simulink model "addTw_mdl5"  (R2014a)
settings: Solver=FixedStepDiscrete  SolverMode=SingleTasking  StartTime=TIME(1)  StopTime=TIME(end)  FixedStep=SIMSTEP  RelTol=1e-3
model workspace (MAT data in the model file):
  autoc_mdd_data01 : struct (value not decoded)
undefined symbols (not defined in the file or in its folder): map_mr4_01, map_mr4_02, map_mr4_03, map_mr4_04, map_mr4_05, map_mr4_06, map_mr4_07, map_mr4_08, Parameter114, Parameter115, Parameter131, Parameter141, Parameter143, Parameter144, Parameter51, Parameter52, Parameter53, Parameter70, Parameter71, Parameter92, Parameter93, SIMSTEP
(part 3 of 3)

== system addTw_mdl5/SubSystem2611/SubSystem2691/SubSystem2693/SubSystem2695/SubSystem2703 ==
  note: ***編集禁止***
  input : Inport
  element : Inport  Port=2
  Assignment : Assignment  IndexOptions=Index vector (port)  OutputSizes=[1 1]
  Inside_DSR : DataStoreRead  DataStoreName=DSM335
  Inside_DSW : DataStoreWrite  DataStoreName=DSM335
  wires:
  element/1 -> Assignment/3
  input/1 -> Assignment/2
  Inside_DSR/1 -> Assignment/1
  Assignment/1 -> Inside_DSW/1

== system addTw_mdl5/SubSystem2611/SubSystem2691/SubSystem2693/SubSystem2695/SubSystem2704 ==
  note: ***編集禁止***
  input : Inport
  element : Inport  Port=2
  Assignment : Assignment  IndexOptions=Index vector (port)  OutputSizes=[1 1]
  Inside_DSR : DataStoreRead  DataStoreName=DSM348
  Inside_DSW : DataStoreWrite  DataStoreName=DSM348
  wires:
  Assignment/1 -> Inside_DSW/1
  Inside_DSR/1 -> Assignment/1
  input/1 -> Assignment/2
  element/1 -> Assignment/3

== system addTw_mdl5/SubSystem2611/SubSystem2691/SubSystem2693/SubSystem2695/SubSystem2705 ==
  note: ***編集禁止***
  input : Inport
  element : Inport  Port=2
  Assignment : Assignment  IndexOptions=Index vector (port)  OutputSizes=[1 1]
  Inside_DSR : DataStoreRead  DataStoreName=DSM349
  Inside_DSW : DataStoreWrite  DataStoreName=DSM349
  wires:
  Assignment/1 -> Inside_DSW/1
  Inside_DSR/1 -> Assignment/1
  input/1 -> Assignment/2
  element/1 -> Assignment/3

== system addTw_mdl5/SubSystem2611/SubSystem2691/SubSystem2693/SubSystem2695/SubSystem2706 ==
  note: ***編集禁止***
  input : Inport
  element : Inport  Port=2
  Assignment : Assignment  IndexOptions=Index vector (port)  OutputSizes=[1 1]
  Inside_DSR : DataStoreRead  DataStoreName=DSM347
  Inside_DSW : DataStoreWrite  DataStoreName=DSM347
  wires:
  Assignment/1 -> Inside_DSW/1
  Inside_DSR/1 -> Assignment/1
  input/1 -> Assignment/2
  element/1 -> Assignment/3

== system addTw_mdl5/SubSystem2611/SubSystem2612/SubSystem2620/SubSystem2624/SubSystem2627/SubSystem2628 ==
  note: ***編集禁止***
  element : Inport
  Inside_DSR : DataStoreRead  DataStoreName=DSM147
  Selector : Selector  IndexOptions=Index vector (port)  Indices=[1 3]
  Output : Outport
  wires:
  Selector/1 -> Output/1
  element/1 -> Selector/2
  Inside_DSR/1 -> Selector/1

== system addTw_mdl5/SubSystem2611/SubSystem2612/SubSystem2620/SubSystem2624/SubSystem2627/SubSystem2629 ==
  note: ***編集禁止***
  element : Inport
  Inside_DSR : DataStoreRead  DataStoreName=DSM304
  Selector : Selector  IndexOptions=Index vector (port)  Indices=[1 3]
  Output : Outport
  wires:
  Inside_DSR/1 -> Selector/1
  element/1 -> Selector/2
  Selector/1 -> Output/1

== system addTw_mdl5/SubSystem2611/SubSystem2612/SubSystem2620/SubSystem2624/SubSystem2627/SubSystem2630 ==
  note: ***編集禁止***
  element : Inport
  Inside_DSR : DataStoreRead  DataStoreName=DSM346
  Selector : Selector  IndexOptions=Index vector (port)  Indices=[1 3]
  Output : Outport
  wires:
  Selector/1 -> Output/1
  element/1 -> Selector/2
  Inside_DSR/1 -> Selector/1

== system addTw_mdl5/SubSystem2611/SubSystem2612/SubSystem2620/SubSystem2624/SubSystem2627/SubSystem2631 ==
  note: ***編集禁止***
  input : Inport
  element : Inport  Port=2
  Assignment : Assignment  IndexOptions=Index vector (port)  OutputSizes=[1 1]
  Inside_DSR : DataStoreRead  DataStoreName=DSM346
  Inside_DSW : DataStoreWrite  DataStoreName=DSM346
  wires:
  Assignment/1 -> Inside_DSW/1
  Inside_DSR/1 -> Assignment/1
  input/1 -> Assignment/2
  element/1 -> Assignment/3

== system addTw_mdl5/SubSystem2611/SubSystem2612/SubSystem2620/SubSystem2624/SubSystem2627/SubSystem2632 ==
  note: ***編集禁止***
  input : Inport
  element : Inport  Port=2
  Assignment : Assignment  IndexOptions=Index vector (port)  OutputSizes=[1 1]
  Inside_DSR : DataStoreRead  DataStoreName=DSM349
  Inside_DSW : DataStoreWrite  DataStoreName=DSM349
  wires:
  Assignment/1 -> Inside_DSW/1
  Inside_DSR/1 -> Assignment/1
  input/1 -> Assignment/2
  element/1 -> Assignment/3

== system addTw_mdl5/SubSystem2611/SubSystem2612/SubSystem2620/SubSystem2624/SubSystem2627/SubSystem2633 ==
  note: ***編集禁止***
  input : Inport
  element : Inport  Port=2
  Assignment : Assignment  IndexOptions=Index vector (port)  OutputSizes=[1 1]
  Inside_DSR : DataStoreRead  DataStoreName=DSM348
  Inside_DSW : DataStoreWrite  DataStoreName=DSM348
  wires:
  element/1 -> Assignment/3
  input/1 -> Assignment/2
  Inside_DSR/1 -> Assignment/1
  Assignment/1 -> Inside_DSW/1

== system addTw_mdl5/SubSystem2611/SubSystem2612/SubSystem2620/SubSystem2624/SubSystem2627/SubSystem2634 ==
  note: ***編集禁止***
  input : Inport
  element : Inport  Port=2
  Assignment : Assignment  IndexOptions=Index vector (port)  OutputSizes=[1 1]
  Inside_DSR : DataStoreRead  DataStoreName=DSM347
  Inside_DSW : DataStoreWrite  DataStoreName=DSM347
  wires:
  element/1 -> Assignment/3
  input/1 -> Assignment/2
  Inside_DSR/1 -> Assignment/1
  Assignment/1 -> Inside_DSW/1

== system addTw_mdl5/SubSystem2611/SubSystem2612/SubSystem2620/SubSystem2624/SubSystem2627/SubSystem2635 ==
  note: ***編集禁止***
  In1 : Inport
  In2 : Inport  Port=2
  RO1 : RelationalOperator  Operator===  InputSameDT=on
  single1 : DataTypeConversion  OutDataTypeStr=single  SaturateOnIntegerOverflow=on  RndMeth=Zero
  single2 : DataTypeConversion  OutDataTypeStr=single  SaturateOnIntegerOverflow=on  RndMeth=Zero
  Out1 : Outport
  wires:
  single2/1 -> RO1/2
  single1/1 -> RO1/1
  In1/1 -> single1/1
  In2/1 -> single2/1
  RO1/1 -> Out1/1

== system addTw_mdl5/SubSystem2611/SubSystem2612/SubSystem2620/SubSystem2624/SubSystem2638/SubSystem2639 ==
  note: ***編集禁止***
  element : Inport
  Inside_DSR : DataStoreRead  DataStoreName=DSM97
  Selector : Selector  IndexOptions=Index vector (port)  Indices=[1 3]
  Output : Outport
  wires:
  Inside_DSR/1 -> Selector/1
  element/1 -> Selector/2
  Selector/1 -> Output/1

== system addTw_mdl5/SubSystem2611/SubSystem2612/SubSystem2620/SubSystem2624/SubSystem2638/SubSystem2640 ==
  note: ***編集禁止***
  element : Inport
  Inside_DSR : DataStoreRead  DataStoreName=DSM318
  Selector : Selector  IndexOptions=Index vector (port)  Indices=[1 3]
  Output : Outport
  wires:
  Selector/1 -> Output/1
  element/1 -> Selector/2
  Inside_DSR/1 -> Selector/1

== system addTw_mdl5/SubSystem2611/SubSystem2612/SubSystem2620/SubSystem2624/SubSystem2638/SubSystem2641 ==
  note: ***編集禁止***
  mult : Inport
  div : Inport  Port=2
  Product : Product  Inputs=*/  SaturateOnIntegerOverflow=on  RndMeth=Zero  InputSameDT=on  OutDataTypeStr=Inherit: Same as first input
  Out : Outport
  wires:
  div/1 -> Product/2
  mult/1 -> Product/1
  Product/1 -> Out/1

== system addTw_mdl5/SubSystem2611/SubSystem2612/SubSystem2620/SubSystem2624/SubSystem2638/SubSystem2642 ==
  note: ***編集禁止***
  mult : Inport
  div : Inport  Port=2
  Product : Product  Inputs=*/  SaturateOnIntegerOverflow=on  RndMeth=Zero  InputSameDT=on  OutDataTypeStr=Inherit: Same as first input
  Out : Outport
  wires:
  Product/1 -> Out/1
  mult/1 -> Product/1
  div/1 -> Product/2

== system addTw_mdl5/SubSystem2611/SubSystem2612/SubSystem2620/SubSystem2624/SubSystem2638/SubSystem2643 ==
  note: ***編集禁止***
  Max : Inport
  Input : Inport  Port=2
  Min1 : MinMax  Inputs=2  SaturateOnIntegerOverflow=on  InputSameDT=on
  Output : Outport
  wires:
  Max/1 -> Min1/1
  Input/1 -> Min1/2
  Min1/1 -> Output/1

== system addTw_mdl5/SubSystem2611/SubSystem2612/SubSystem2620/SubSystem2624/SubSystem2644/SubSystem2645 ==
  note: ***編集禁止***
  element : Inport
  Inside_DSR : DataStoreRead  DataStoreName=DSM115
  Selector : Selector  IndexOptions=Index vector (port)  Indices=[1 3]
  Output : Outport
  wires:
  Inside_DSR/1 -> Selector/1
  element/1 -> Selector/2
  Selector/1 -> Output/1

== system addTw_mdl5/SubSystem2611/SubSystem2612/SubSystem2620/SubSystem2624/SubSystem2644/SubSystem2646 ==
  note: ***編集禁止***
  element : Inport
  Inside_DSR : DataStoreRead  DataStoreName=DSM119
  Selector : Selector  IndexOptions=Index vector (port)  Indices=[1 3]
  Output : Outport
  wires:
  Selector/1 -> Output/1
  element/1 -> Selector/2
  Inside_DSR/1 -> Selector/1

== system addTw_mdl5/SubSystem2611/SubSystem2612/SubSystem2620/SubSystem2624/SubSystem2644/SubSystem2647 ==
  note: ***編集禁止***
  element : Inport
  Inside_DSR : DataStoreRead  DataStoreName=DSM102
  Selector : Selector  IndexOptions=Index vector (port)  Indices=[1 3]
  Output : Outport
  wires:
  Selector/1 -> Output/1
  element/1 -> Selector/2
  Inside_DSR/1 -> Selector/1

== system addTw_mdl5/SubSystem2611/SubSystem2612/SubSystem2620/SubSystem2624/SubSystem2644/SubSystem2648 ==
  note: ***編集禁止***
  element : Inport
  Inside_DSR : DataStoreRead  DataStoreName=DSM104
  Selector : Selector  IndexOptions=Index vector (port)  Indices=[1 3]
  Output : Outport
  wires:
  Inside_DSR/1 -> Selector/1
  element/1 -> Selector/2
  Selector/1 -> Output/1

== system addTw_mdl5/SubSystem2611/SubSystem2612/SubSystem2620/SubSystem2624/SubSystem2644/SubSystem2649 ==
  note: ***編集禁止***
  element : Inport
  Inside_DSR : DataStoreRead  DataStoreName=DSM110
  Selector : Selector  IndexOptions=Index vector (port)  Indices=[1 3]
  Output : Outport
  wires:
  Inside_DSR/1 -> Selector/1
  element/1 -> Selector/2
  Selector/1 -> Output/1

== system addTw_mdl5/SubSystem2611/SubSystem2612/SubSystem2620/SubSystem2624/SubSystem2644/SubSystem2650 ==
  note: ***編集禁止***
  element : Inport
  Inside_DSR : DataStoreRead  DataStoreName=DSM112
  Selector : Selector  IndexOptions=Index vector (port)  Indices=[1 3]
  Output : Outport
  wires:
  Selector/1 -> Output/1
  element/1 -> Selector/2
  Inside_DSR/1 -> Selector/1

== system addTw_mdl5/SubSystem2611/SubSystem2612/SubSystem2620/SubSystem2624/SubSystem2644/SubSystem2651 ==
  note: ***編集禁止***
  element : Inport
  Inside_DSR : DataStoreRead  DataStoreName=DSM116
  Selector : Selector  IndexOptions=Index vector (port)  Indices=[1 3]
  Output : Outport
  wires:
  Selector/1 -> Output/1
  element/1 -> Selector/2
  Inside_DSR/1 -> Selector/1

== system addTw_mdl5/SubSystem2611/SubSystem2612/SubSystem2620/SubSystem2624/SubSystem2644/SubSystem2652 ==
  note: ***編集禁止***
  element : Inport
  Inside_DSR : DataStoreRead  DataStoreName=DSM120
  Selector : Selector  IndexOptions=Index vector (port)  Indices=[1 3]
  Output : Outport
  wires:
  Inside_DSR/1 -> Selector/1
  element/1 -> Selector/2
  Selector/1 -> Output/1

== system addTw_mdl5/SubSystem2611/SubSystem2612/SubSystem2620/SubSystem2624/SubSystem2644/SubSystem2653 ==
  note: ***編集禁止***
  element : Inport
  Inside_DSR : DataStoreRead  DataStoreName=DSM122
  Selector : Selector  IndexOptions=Index vector (port)  Indices=[1 3]
  Output : Outport
  wires:
  Inside_DSR/1 -> Selector/1
  element/1 -> Selector/2
  Selector/1 -> Output/1

== system addTw_mdl5/SubSystem2611/SubSystem2612/SubSystem2620/SubSystem2624/SubSystem2644/SubSystem2654 ==
  note: ***編集禁止***
  element : Inport
  Inside_DSR : DataStoreRead  DataStoreName=DSM125
  Selector : Selector  IndexOptions=Index vector (port)  Indices=[1 3]
  Output : Outport
  wires:
  Selector/1 -> Output/1
  element/1 -> Selector/2
  Inside_DSR/1 -> Selector/1

== system addTw_mdl5/SubSystem2611/SubSystem2612/SubSystem2620/SubSystem2624/SubSystem2644/SubSystem2655 ==
  note: ***編集禁止***
  element : Inport
  Inside_DSR : DataStoreRead  DataStoreName=DSM123
  Selector : Selector  IndexOptions=Index vector (port)  Indices=[1 3]
  Output : Outport
  wires:
  Selector/1 -> Output/1
  element/1 -> Selector/2
  Inside_DSR/1 -> Selector/1

== system addTw_mdl5/SubSystem2611/SubSystem2612/SubSystem2620/SubSystem2624/SubSystem2644/SubSystem2656 ==
  note: ***編集禁止***
  element : Inport
  Inside_DSR : DataStoreRead  DataStoreName=DSM126
  Selector : Selector  IndexOptions=Index vector (port)  Indices=[1 3]
  Output : Outport
  wires:
  Inside_DSR/1 -> Selector/1
  element/1 -> Selector/2
  Selector/1 -> Output/1

== system addTw_mdl5/SubSystem2611/SubSystem2612/SubSystem2620/SubSystem2624/SubSystem2644/SubSystem2657 ==
  note: ***編集禁止***
  element : Inport
  Inside_DSR : DataStoreRead  DataStoreName=DSM106
  Selector : Selector  IndexOptions=Index vector (port)  Indices=[1 3]
  Output : Outport
  wires:
  Inside_DSR/1 -> Selector/1
  element/1 -> Selector/2
  Selector/1 -> Output/1

== system addTw_mdl5/SubSystem2611/SubSystem2612/SubSystem2620/SubSystem2624/SubSystem2644/SubSystem2658 ==
  note: ***編集禁止***
  element : Inport
  Inside_DSR : DataStoreRead  DataStoreName=DSM108
  Selector : Selector  IndexOptions=Index vector (port)  Indices=[1 3]
  Output : Outport
  wires:
  Selector/1 -> Output/1
  element/1 -> Selector/2
  Inside_DSR/1 -> Selector/1

== system addTw_mdl5/SubSystem2611/SubSystem2612/SubSystem2620/SubSystem2624/SubSystem2644/SubSystem2659 ==
  note: ***編集禁止***
  In1 : Inport
  In2 : Inport  Port=2
  RO1 : RelationalOperator  Operator===  InputSameDT=on
  single1 : DataTypeConversion  OutDataTypeStr=single  SaturateOnIntegerOverflow=on  RndMeth=Zero
  single2 : DataTypeConversion  OutDataTypeStr=single  SaturateOnIntegerOverflow=on  RndMeth=Zero
  Out1 : Outport
  wires:
  single2/1 -> RO1/2
  single1/1 -> RO1/1
  In1/1 -> single1/1
  In2/1 -> single2/1
  RO1/1 -> Out1/1

== system addTw_mdl5/SubSystem2611/SubSystem2612/SubSystem2620/SubSystem2624/SubSystem2644/SubSystem2660 ==
  note: ***編集禁止***
  In1 : Inport
  In2 : Inport  Port=2
  RO1 : RelationalOperator  Operator===  InputSameDT=on
  single1 : DataTypeConversion  OutDataTypeStr=single  SaturateOnIntegerOverflow=on  RndMeth=Zero
  single2 : DataTypeConversion  OutDataTypeStr=single  SaturateOnIntegerOverflow=on  RndMeth=Zero
  Out1 : Outport
  wires:
  RO1/1 -> Out1/1
  In2/1 -> single2/1
  In1/1 -> single1/1
  single1/1 -> RO1/1
  single2/1 -> RO1/2

== system addTw_mdl5/SubSystem2611/SubSystem2612/SubSystem2620/SubSystem2624/SubSystem2644/SubSystem2661 ==
  note: ***編集禁止***
  In1 : Inport
  In2 : Inport  Port=2
  RO1 : RelationalOperator  Operator===  InputSameDT=on
  single1 : DataTypeConversion  OutDataTypeStr=single  SaturateOnIntegerOverflow=on  RndMeth=Zero
  single2 : DataTypeConversion  OutDataTypeStr=single  SaturateOnIntegerOverflow=on  RndMeth=Zero
  Out1 : Outport
  wires:
  single2/1 -> RO1/2
  single1/1 -> RO1/1
  In1/1 -> single1/1
  In2/1 -> single2/1
  RO1/1 -> Out1/1

== system addTw_mdl5/SubSystem2611/SubSystem2612/SubSystem2620/SubSystem2624/SubSystem2644/SubSystem2662 ==
  note: ***編集禁止***
  In1 : Inport
  In2 : Inport  Port=2
  RO1 : RelationalOperator  Operator===  InputSameDT=on
  single1 : DataTypeConversion  OutDataTypeStr=single  SaturateOnIntegerOverflow=on  RndMeth=Zero
  single2 : DataTypeConversion  OutDataTypeStr=single  SaturateOnIntegerOverflow=on  RndMeth=Zero
  Out1 : Outport
  wires:
  RO1/1 -> Out1/1
  In2/1 -> single2/1
  In1/1 -> single1/1
  single1/1 -> RO1/1
  single2/1 -> RO1/2

== system addTw_mdl5/SubSystem2611/SubSystem2612/SubSystem2620/SubSystem2624/SubSystem2644/SubSystem2663 ==
  note: ***編集禁止***
  In1 : Inport
  In2 : Inport  Port=2
  RO1 : RelationalOperator  Operator===  InputSameDT=on
  single1 : DataTypeConversion  OutDataTypeStr=single  SaturateOnIntegerOverflow=on  RndMeth=Zero
  single2 : DataTypeConversion  OutDataTypeStr=single  SaturateOnIntegerOverflow=on  RndMeth=Zero
  Out1 : Outport
  wires:
  RO1/1 -> Out1/1
  In2/1 -> single2/1
  In1/1 -> single1/1
  single1/1 -> RO1/1
  single2/1 -> RO1/2

== system addTw_mdl5/SubSystem2611/SubSystem2612/SubSystem2620/SubSystem2624/SubSystem2644/SubSystem2664 ==
  note: ***編集禁止***
  In1 : Inport
  In2 : Inport  Port=2
  RO1 : RelationalOperator  Operator===  InputSameDT=on
  single1 : DataTypeConversion  OutDataTypeStr=single  SaturateOnIntegerOverflow=on  RndMeth=Zero
  single2 : DataTypeConversion  OutDataTypeStr=single  SaturateOnIntegerOverflow=on  RndMeth=Zero
  Out1 : Outport
  wires:
  RO1/1 -> Out1/1
  In2/1 -> single2/1
  In1/1 -> single1/1
  single1/1 -> RO1/1
  single2/1 -> RO1/2

== system addTw_mdl5/SubSystem2611/SubSystem2612/SubSystem2665/SubSystem2666/SubSystem2670/SubSystem2671 ==
  note: ***編集禁止***
  element : Inport
  Inside_DSR : DataStoreRead  DataStoreName=DSM97
  Selector : Selector  IndexOptions=Index vector (port)  Indices=[1 3]
  Output : Outport
  wires:
  Inside_DSR/1 -> Selector/1
  element/1 -> Selector/2
  Selector/1 -> Output/1

== system addTw_mdl5/SubSystem2611/SubSystem2612/SubSystem2665/SubSystem2666/SubSystem2670/SubSystem2672 ==
  note: ***編集禁止***
  element : Inport
  Inside_DSR : DataStoreRead  DataStoreName=DSM318
  Selector : Selector  IndexOptions=Index vector (port)  Indices=[1 3]
  Output : Outport
  wires:
  Selector/1 -> Output/1
  element/1 -> Selector/2
  Inside_DSR/1 -> Selector/1

== system addTw_mdl5/SubSystem2611/SubSystem2612/SubSystem2665/SubSystem2666/SubSystem2670/SubSystem2673 ==
  note: ***編集禁止***
  element : Inport
  Inside_DSR : DataStoreRead  DataStoreName=DSM36
  Selector : Selector  IndexOptions=Index vector (port)  Indices=[1 3]
  Output : Outport
  wires:
  Inside_DSR/1 -> Selector/1
  element/1 -> Selector/2
  Selector/1 -> Output/1

== system addTw_mdl5/SubSystem2611/SubSystem2612/SubSystem2665/SubSystem2666/SubSystem2670/SubSystem2674 ==
  note: ***編集禁止***
  input : Inport
  element : Inport  Port=2
  Assignment : Assignment  IndexOptions=Index vector (port)  OutputSizes=[1 1]
  Inside_DSR : DataStoreRead  DataStoreName=DSM321
  Inside_DSW : DataStoreWrite  DataStoreName=DSM321
  wires:
  element/1 -> Assignment/3
  input/1 -> Assignment/2
  Inside_DSR/1 -> Assignment/1
  Assignment/1 -> Inside_DSW/1

== system addTw_mdl5/SubSystem2611/SubSystem2612/SubSystem2665/SubSystem2666/SubSystem2670/SubSystem2675 ==
  note: ***編集禁止***
  In1 : Inport
  In2 : Inport  Port=2
  RO1 : RelationalOperator  Operator===  InputSameDT=on
  single1 : DataTypeConversion  OutDataTypeStr=single  SaturateOnIntegerOverflow=on  RndMeth=Zero
  single2 : DataTypeConversion  OutDataTypeStr=single  SaturateOnIntegerOverflow=on  RndMeth=Zero
  Out1 : Outport
  wires:
  single2/1 -> RO1/2
  single1/1 -> RO1/1
  In1/1 -> single1/1
  In2/1 -> single2/1
  RO1/1 -> Out1/1

== system addTw_mdl5/SubSystem2611/SubSystem2612/SubSystem2665/SubSystem2666/SubSystem2676/SubSystem2677 ==
  note: ***編集禁止***
  element : Inport
  Inside_DSR : DataStoreRead  DataStoreName=DSM334
  Selector : Selector  IndexOptions=Index vector (port)  Indices=[1 3]
  Output : Outport
  wires:
  Inside_DSR/1 -> Selector/1
  element/1 -> Selector/2
  Selector/1 -> Output/1

== system addTw_mdl5/SubSystem2611/SubSystem2612/SubSystem2665/SubSystem2666/SubSystem2676/SubSystem2678 ==
  note: ***編集禁止***
  element : Inport
  Inside_DSR : DataStoreRead  DataStoreName=DSM335
  Selector : Selector  IndexOptions=Index vector (port)  Indices=[1 3]
  Output : Outport
  wires:
  Selector/1 -> Output/1
  element/1 -> Selector/2
  Inside_DSR/1 -> Selector/1

== system addTw_mdl5/SubSystem2611/SubSystem2612/SubSystem2665/SubSystem2666/SubSystem2676/SubSystem2679 ==
  note: ***編集禁止***
  element : Inport
  Inside_DSR : DataStoreRead  DataStoreName=DSM336
  Selector : Selector  IndexOptions=Index vector (port)  Indices=[1 3]
  Output : Outport
  wires:
  Inside_DSR/1 -> Selector/1
  element/1 -> Selector/2
  Selector/1 -> Output/1

== system addTw_mdl5/SubSystem2611/SubSystem2612/SubSystem2665/SubSystem2666/SubSystem2676/SubSystem2680 ==
  note: ***編集禁止***
  element : Inport
  Inside_DSR : DataStoreRead  DataStoreName=DSM337
  Selector : Selector  IndexOptions=Index vector (port)  Indices=[1 3]
  Output : Outport
  wires:
  Selector/1 -> Output/1
  element/1 -> Selector/2
  Inside_DSR/1 -> Selector/1

== system addTw_mdl5/SubSystem2611/SubSystem2612/SubSystem2665/SubSystem2666/SubSystem2676/SubSystem2681 ==
  note: ***編集禁止***
  input : Inport
  element : Inport  Port=2
  Assignment : Assignment  IndexOptions=Index vector (port)  OutputSizes=[1 1]
  Inside_DSR : DataStoreRead  DataStoreName=DSM334
  Inside_DSW : DataStoreWrite  DataStoreName=DSM334
  wires:
  Assignment/1 -> Inside_DSW/1
  Inside_DSR/1 -> Assignment/1
  input/1 -> Assignment/2
  element/1 -> Assignment/3

== system addTw_mdl5/SubSystem2611/SubSystem2612/SubSystem2665/SubSystem2666/SubSystem2676/SubSystem2682 ==
  note: ***編集禁止***
  input : Inport
  element : Inport  Port=2
  Assignment : Assignment  IndexOptions=Index vector (port)  OutputSizes=[1 1]
  Inside_DSR : DataStoreRead  DataStoreName=DSM335
  Inside_DSW : DataStoreWrite  DataStoreName=DSM335
  wires:
  element/1 -> Assignment/3
  input/1 -> Assignment/2
  Inside_DSR/1 -> Assignment/1
  Assignment/1 -> Inside_DSW/1

== system addTw_mdl5/SubSystem2611/SubSystem2612/SubSystem2665/SubSystem2666/SubSystem2676/SubSystem2683 ==
  note: ***編集禁止***
  input : Inport
  element : Inport  Port=2
  Assignment : Assignment  IndexOptions=Index vector (port)  OutputSizes=[1 1]
  Inside_DSR : DataStoreRead  DataStoreName=DSM336
  Inside_DSW : DataStoreWrite  DataStoreName=DSM336
  wires:
  Assignment/1 -> Inside_DSW/1
  Inside_DSR/1 -> Assignment/1
  input/1 -> Assignment/2
  element/1 -> Assignment/3

== system addTw_mdl5/SubSystem2611/SubSystem2612/SubSystem2665/SubSystem2666/SubSystem2676/SubSystem2684 ==
  note: ***編集禁止***
  input : Inport
  element : Inport  Port=2
  Assignment : Assignment  IndexOptions=Index vector (port)  OutputSizes=[1 1]
  Inside_DSR : DataStoreRead  DataStoreName=DSM337
  Inside_DSW : DataStoreWrite  DataStoreName=DSM337
  wires:
  element/1 -> Assignment/3
  input/1 -> Assignment/2
  Inside_DSR/1 -> Assignment/1
  Assignment/1 -> Inside_DSW/1

== system addTw_mdl5/SubSystem2611/SubSystem2612/SubSystem2665/SubSystem2666/SubSystem2676/SubSystem2685 ==
  note: ***編集禁止***
  In1 : Inport
  In2 : Inport  Port=2
  RO1 : RelationalOperator  Operator===  InputSameDT=on
  single1 : DataTypeConversion  OutDataTypeStr=single  SaturateOnIntegerOverflow=on  RndMeth=Zero
  single2 : DataTypeConversion  OutDataTypeStr=single  SaturateOnIntegerOverflow=on  RndMeth=Zero
  Out1 : Outport
  wires:
  RO1/1 -> Out1/1
  In2/1 -> single2/1
  In1/1 -> single1/1
  single1/1 -> RO1/1
  single2/1 -> RO1/2

== system addTw_mdl5/SubSystem2611/SubSystem2612/SubSystem2665/SubSystem2666/SubSystem2676/SubSystem2686 ==
  note: ***編集禁止***
  In1 : Inport
  In2 : Inport  Port=2
  RO1 : RelationalOperator  Operator===  InputSameDT=on
  single1 : DataTypeConversion  OutDataTypeStr=single  SaturateOnIntegerOverflow=on  RndMeth=Zero
  single2 : DataTypeConversion  OutDataTypeStr=single  SaturateOnIntegerOverflow=on  RndMeth=Zero
  Out1 : Outport
  wires:
  RO1/1 -> Out1/1
  In2/1 -> single2/1
  In1/1 -> single1/1
  single1/1 -> RO1/1
  single2/1 -> RO1/2

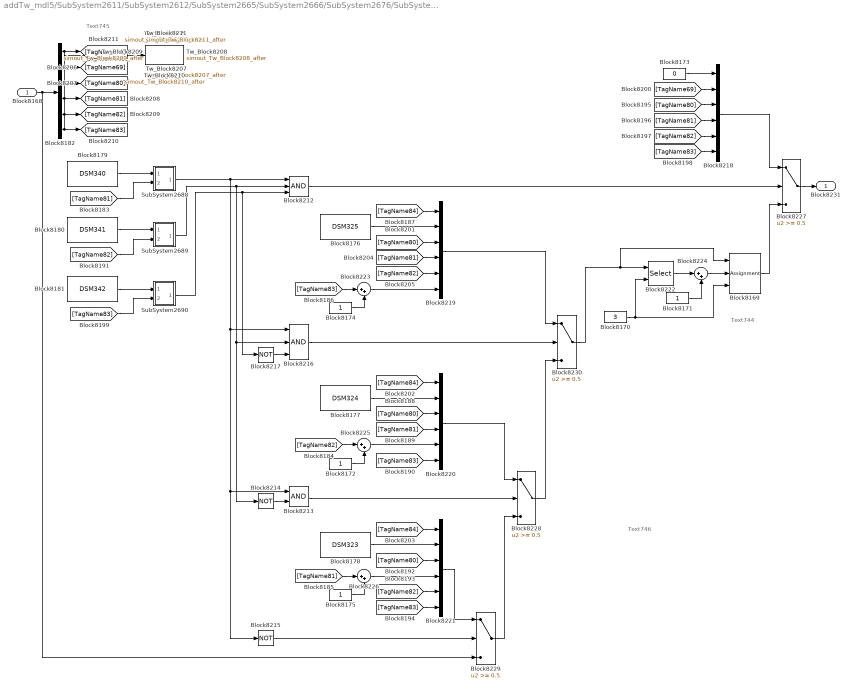
== system addTw_mdl5/SubSystem2611/SubSystem2612/SubSystem2665/SubSystem2666/SubSystem2676/SubSystem2687 ==
  note: Text746
  note: Text745
  note: Text744
  Block8168 : Inport
  Block8169 : Assignment  IndexOptions=Index vector (port)  OutputSizes=[1 1]
  Block8170 : Constant  Value=3  OutDataTypeStr=double  SampleTime=-1
  Block{8171..8172,8174..8175} (4 alike) : Constant  OutDataTypeStr=double  SampleTime=-1
  Block8173 : Constant  Value=0  OutDataTypeStr=double  SampleTime=-1
  Block8176 : DataStoreRead  DataStoreName=DSM325
  Block8177 : DataStoreRead  DataStoreName=DSM324
  Block8178 : DataStoreRead  DataStoreName=DSM323
  Block8179 : DataStoreRead  DataStoreName=DSM340
  Block8180 : DataStoreRead  DataStoreName=DSM341
  Block8181 : DataStoreRead  DataStoreName=DSM342
  Block8182 : Demux  Outputs=6
  Block8212 : Logic  Inputs=3
  Block8213 : Logic
  Block8214 : Logic  Operator=NOT
  Block8215 : Logic  Operator=NOT
  Block8216 : Logic  Inputs=3
  Block8217 : Logic  Operator=NOT
  Block{8218..8221} (4 alike) : Mux  Inputs=6
  Block8222 : Selector  IndexOptions=Index vector (port)  Indices=[1 3]
  Block{8223..8226} (4 alike) : Sum  Inputs=|++  OutDataTypeStr=double  RndMeth=Zero  SaturateOnIntegerOverflow=on  InputSameDT=on
  Block{8227..8230} (4 alike) : Switch  Threshold=0.5  RndMeth=Zero  SaturateOnIntegerOverflow=on  InputSameDT=on
  SubSystem2688 : Subsystem
  SubSystem2689 : Subsystem
  SubSystem2690 : Subsystem
  Tw_Block8206 : ToWorkspace  VariableName=simout_Tw_Block8206_after  SaveFormat=Timeseries  SampleTime=-1
  Tw_Block8207 : ToWorkspace  VariableName=simout_Tw_Block8207_after  SaveFormat=Timeseries  SampleTime=-1
  Tw_Block8208 : ToWorkspace  VariableName=simout_Tw_Block8208_after  SaveFormat=Timeseries  SampleTime=-1
  Tw_Block8209 : ToWorkspace  VariableName=simout_Tw_Block8209_after  SaveFormat=Timeseries  SampleTime=-1
  Tw_Block8210 : ToWorkspace  VariableName=simout_Tw_Block8210_after  SaveFormat=Timeseries  SampleTime=-1
  Tw_Block8211 : ToWorkspace  VariableName=simout_Tw_Block8211_after  SaveFormat=Timeseries  SampleTime=-1
  Block8231 : Outport
  wires:
  SubSystem2688/1(Out1) -> Block8212/1, Block8216/1, Block8213/1, Block8215/1
  SubSystem2689/1(Out1) -> Block8212/2, Block8216/2, Block8214/1
  SubSystem2690/1(Out1) -> Block8212/3, Block8217/1
  Block8212/1 -> Block8227/2
  Block8213/1 -> Block8228/2
  Block8215/1 -> Block8229/2
  Block8218/1 -> Block8227/1
  Block8179/1 -> SubSystem2688/1(In1)
  Block8180/1 -> SubSystem2689/1(In1)
  Block8181/1 -> SubSystem2690/1(In1)
  [TagName81] -> SubSystem2688/2(In2)
  [TagName82] -> SubSystem2689/2(In2)
  [TagName83] -> SubSystem2690/2(In2)
  Block8216/1 -> Block8230/2
  Block8219/1 -> Block8230/1
  Block8220/1 -> Block8228/1
  Block8221/1 -> Block8229/1
  Block8228/1 -> Block8230/3
  Block8229/1 -> Block8228/3
  Block8217/1 -> Block8216/3
  Block8214/1 -> Block8213/2
  Block8227/1 -> Block8231/1
  Block8173/1 -> Block8218/1
  [TagName69] -> Block8218/2
  [TagName80] -> Block8218/3
  [TagName81] -> Block8218/4
  [TagName82] -> Block8218/5
  [TagName83] -> Block8218/6
  [TagName84] -> Block8219/1
  [TagName80] -> Block8219/3
  [TagName81] -> Block8219/4
  [TagName82] -> Block8219/5
  Block8174/1 -> Block8223/2
  Block8176/1 -> Block8219/2
  Block8223/1 -> Block8219/6
  [TagName83] -> Block8223/1
  Block8169/1 -> Block8227/3
  Block8171/1 -> Block8224/2
  Block8224/1 -> Block8169/2
  Block8222/1 -> Block8224/1
  Block8170/1 -> Block8169/3, Block8222/2
  Block8230/1 -> Block8222/1, Block8169/1
  [TagName84] -> Block8220/1
  [TagName80] -> Block8220/3
  [TagName81] -> Block8220/4
  Block8225/1 -> Block8220/5
  Block8172/1 -> Block8225/2
  Block8177/1 -> Block8220/2
  [TagName83] -> Block8220/6
  [TagName82] -> Block8225/1
  [TagName84] -> Block8221/1
  [TagName80] -> Block8221/3
  Block8178/1 -> Block8221/2
  [TagName83] -> Block8221/6
  [TagName82] -> Block8221/5
  Block8226/1 -> Block8221/4
  Block8175/1 -> Block8226/2
  [TagName81] -> Block8226/1
  Block8182/1 -> [TagName84], Tw_Block8211/1
  Block8182/2 -> [TagName69], Tw_Block8206/1
  Block8182/3 -> [TagName80], Tw_Block8207/1
  Block8182/4 -> [TagName81], Tw_Block8208/1
  Block8182/5 -> [TagName82], Tw_Block8209/1
  Block8182/6 -> [TagName83], Tw_Block8210/1
  Block8168/1 -> Block8182/1, Block8229/3

== system addTw_mdl5/SubSystem2611/SubSystem2612/SubSystem2665/SubSystem2666/SubSystem2676/SubSystem2687/SubSystem2688 ==
  note: ***編集禁止***
  In1 : Inport
  In2 : Inport  Port=2
  RO1 : RelationalOperator  Operator===  InputSameDT=on
  single1 : DataTypeConversion  OutDataTypeStr=single  SaturateOnIntegerOverflow=on  RndMeth=Zero
  single2 : DataTypeConversion  OutDataTypeStr=single  SaturateOnIntegerOverflow=on  RndMeth=Zero
  Out1 : Outport
  wires:
  RO1/1 -> Out1/1
  In2/1 -> single2/1
  In1/1 -> single1/1
  single1/1 -> RO1/1
  single2/1 -> RO1/2

== system addTw_mdl5/SubSystem2611/SubSystem2612/SubSystem2665/SubSystem2666/SubSystem2676/SubSystem2687/SubSystem2689 ==
  note: ***編集禁止***
  In1 : Inport
  In2 : Inport  Port=2
  RO1 : RelationalOperator  Operator===  InputSameDT=on
  single1 : DataTypeConversion  OutDataTypeStr=single  SaturateOnIntegerOverflow=on  RndMeth=Zero
  single2 : DataTypeConversion  OutDataTypeStr=single  SaturateOnIntegerOverflow=on  RndMeth=Zero
  Out1 : Outport
  wires:
  single2/1 -> RO1/2
  single1/1 -> RO1/1
  In1/1 -> single1/1
  In2/1 -> single2/1
  RO1/1 -> Out1/1

== system addTw_mdl5/SubSystem2611/SubSystem2612/SubSystem2665/SubSystem2666/SubSystem2676/SubSystem2687/SubSystem2690 ==
  note: ***編集禁止***
  In1 : Inport
  In2 : Inport  Port=2
  RO1 : RelationalOperator  Operator===  InputSameDT=on
  single1 : DataTypeConversion  OutDataTypeStr=single  SaturateOnIntegerOverflow=on  RndMeth=Zero
  single2 : DataTypeConversion  OutDataTypeStr=single  SaturateOnIntegerOverflow=on  RndMeth=Zero
  Out1 : Outport
  wires:
  single2/1 -> RO1/2
  single1/1 -> RO1/1
  In1/1 -> single1/1
  In2/1 -> single2/1
  RO1/1 -> Out1/1

== stateflow chart addTw_mdl5/SubSystem2611/SubSystem2691/SubSystem2693/SubSystem2694/For_loop ==
  note: for(i1 = 0; i1 < N_Loop; i1++) {
      |   処理
      | }
  (default) -> (junction 8) : {
      |  idx = 1;
      |  i1 = 0;
      | }
  (junction 11) -> (junction 8) : {i1++;}
  (junction 8) -> (junction 9)
  (junction 10) -> (junction 11) : {
      |  function_call;
      |  idx = idx + 1;
      | }
  (junction 9) -> (junction 10) [order 1] : [i1 < N_Loop]
  (junction 9) -> (junction 12) [order 2]
  data: N_Loop input; i1 local int32; idx output
  events: function_call output FUNCTION_CALL_EVENT
